simulink model "dspafxr_win32"  (Simulink 5.0)
settings: Solver=FixedStepDiscrete  SolverMode=SingleTasking  StartTime=0.0  StopTime=2  RelTol=1e-3  AbsTol=1e-6
PreLoadFcn:
  | load dspafxr;
undefined symbols (not defined in the file or in its folder): fs_afxr
libraries: dspsigops x1, dspsrcs4 x1, dspwin32 x1
Description:
  | Demonstration of audio reverberation for Windows 95/NT only.
settings Model: Creator=don  LastModifiedBy=mkhan  ExtModeTrigMode=oneshot  ExtModeArmWhenConnect=off  SaveTime=off  SaveOutput=off  LimitDataPoints=off  SignalLoggingName=logsOut  IntegerOverflowMsg=none  BlockReductionOpt=off  BooleanDataType=off  ZeroCrossControl=UseLocalSettings  TargetHWChar=2  TargetHWWordLengths=8,16,32,32  RTWMathFcnLibMatFile=iso_c_tmw.mat  RTWOptions="-aEnforceIntegerDowncast=1 -aFoldNonRolledExpr=1 -aInlineInvariantSignals=1 -aInlineParameters=0 -aLocalBlockOutputs=1 -aRollThreshold=2 -aRTWVerbose=1 -aForceParamTrailComments=0 -aGenerateComments=1 -aIgnoreCustomStorageClasses=1 -aIncHierarchyInIds=0 -aMaxRTWIdLen=31 -aShowEliminatedStatements=0 -aReadOnly=0 -aTargetFcnLib=\"iso_c_tmw.mat\" -aIncDataTypeInIds=0 -aPrefixModelToSubsysFcnNames=1 -aInlinedPrmAccess=\"Literals\" -aGenerateFullHeader=1 -aIsPILTarget=0 -aGenerateReport=0 -aLogVarNameModifier=\"rt_\" -aExtMode=0 -aExtModeStaticAlloc=0 -aExtModeTesting=0 -aExtModeStaticAllocSize=1000000 -aExtModeTransport=0"

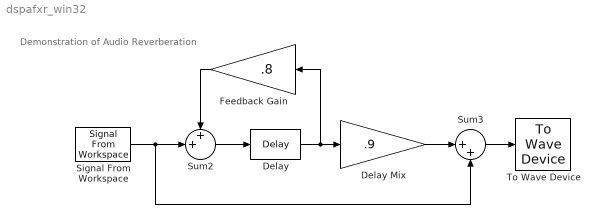
== system dspafxr_win32 ==
  note: Demonstration of
      | Audio Reverberation
  Delay : dspsigops/Delay  dly_unit=Samples  delay=1800  ic_detail=on  dif_ic_for_ch=off  dif_ic_for_dly=off  ic=0  reset_popup=None
  Delay Mix : Gain  Gain=.9  SaturateOnIntegerOverflow=on
  Feedback Gain : Gain  Orientation=left  Gain=.8  SaturateOnIntegerOverflow=on
  Signal From Workspace : dspsrcs4/Signal From Workspace  X=x_afxr  Ts=1/fs_afxr  nsamps=128  OutputAfterFinalValue=Setting to zero
  Sum2 : Sum  Inputs=++|  SaturateOnIntegerOverflow=on  InputSameDT=on
  Sum3 : Sum  Inputs=|++  SaturateOnIntegerOverflow=on  InputSameDT=on
  To Wave Device : dspwin32/To Wave Device  bufDuration=2  initDelay=0.1  useDefaultDevice=on  enable24Bit=off
  wires:
  Signal From Workspace/1 -> Sum3/2, Sum2/2
  Sum2/1 -> Delay/1
  Feedback Gain/1 -> Sum2/1
  Delay/1 -> Feedback Gain/1, Delay Mix/1
  Delay Mix/1 -> Sum3/1
  Sum3/1 -> To Wave Device/1
